simulink library "WECSim_Lib_2019b"  (R2019b)
settings: Solver=ode45  StartTime=0.0  StopTime=10.0  RelTol=1e-3  EnableMultiTasking=on
undefined symbols (not defined in the file or in its folder): body, constraint, mooring, pto, simu, waves, X, Y, Z
libraries: nesl_utility x125, sm_lib x106, $bdroot x16, vrlib x2
(part 9 of 9)

== matlab function WECSim_Lib_2019b/Body Elements/Rigid Body/Hydrodynamic Body/Wave Diffraction and Excitation Force Calculation/Nonlinear FK Force Variant Subsystem/With Nonlinear FroudeKrylov Force/Diffraction and Excitation Forces ==
  data: x input; elv input; center input; f output; tnorm input; area input; rho input; g input; cg input; AH input; w input; dw input; wDepth input; deepWaterWave input; k input; typeNum input; t input; phaseRand input; wp output; wpMeanFS output
function [f, wp, wpMeanFS]  = nonFKForce(x,elv,center,tnorm,area,rho,g,cg,AH,w,dw,wDepth,deepWaterWave,k,typeNum,t,phaseRand)
% Function to calculate the wave excitation force and moment on a
% triangulated surface. The nonlinear excitation forces are calculated by
% intergrating the pressure over the triangulated surface and subtracting
% the linear excitation force (this is added back in later):
%    F_exc_nonlinear = F_exc_total - F_exc_linear
% NOTE: This function assumes that the STL file is imported with its CG at 0,0,0

% Logic to calculate nonFKForce at reduced sample time
[f, wp, wpMeanFS] = calc_force(x,elv,center,tnorm,area,rho,g,cg,AH,w,dw,wDepth,deepWaterWave,k,typeNum,t,phaseRand);
end

function [f, wp, wpMeanFS]  = calc_force(x,elv,center,tnorm,area,rho,g,cg,AH,w,dw,wDepth,deepWaterWave,k,typeNum,t,phaseRand)
% Function to apply translation and rotation, and calculate forces.

% Compute new tri coords after cog rotation and translation
centerMeanFS = offsetXYZ(center,cg);
avMeanFS     = tnorm .* [area area area];

% Compute new tri coords after cog rotation and translation
center = rotateXYZ(center,[1 0 0],x(4));
center = rotateXYZ(center,[0 1 0],x(5));
center = rotateXYZ(center,[0 0 1],x(6));
center = offsetXYZ(center,x);
center = offsetXYZ(center,cg);
% Compute new normal vectors coords after cog rotation and translation
tnorm = rotateXYZ(tnorm,[1 0 0],x(4));
tnorm = rotateXYZ(tnorm,[0 1 0],x(5));
tnorm = rotateXYZ(tnorm,[0 0 1],x(6));

% Copute area vectors
av = tnorm .* [area area area];

% Calculate the free surface
wpMeanFS=pDis(centerMeanFS,       0,AH,w,dw,wDepth,deepWaterWave,t,k,phaseRand,typeNum,rho,g);
wp      =pDis(center      ,     elv,AH,w,dw,wDepth,deepWaterWave,t,k,phaseRand,typeNum,rho,g);

% Calculate forces
f_linear   =FK(centerMeanFS,       cg,avMeanFS,wpMeanFS);
f_nonLinear=FK(center      ,x(1:3)+cg,av      ,wp      );
f = f_nonLinear-f_linear;
end

function f=pDis(center,elv,AH,w,dw,wDepth,deepWaterWave,t,k,phaseRand,typeNum,rho,g)
% Function to calculate pressure distribution
f = zeros(length(center(:,3)),1);
z=zeros(length(center(:,1)),1);
if typeNum <10
elseif typeNum <20
    f = rho.*g.*AH(1).*cos(k(1).*center(:,1)-w(1)*t);
    if deepWaterWave == 0
        z=(center(:,3)-elv).*wDepth./(wDepth+elv);
        f = f.*(cosh(k(1).*(z+wDepth))./cosh(k(1)*wDepth));
    else
        z=(center(:,3)-elv);
        f = f.*exp(k(1).*z);
    end
elseif typeNum <30
    for i=1:length(AH)
        if deepWaterWave == 0 && wDepth <= 0.5*pi/k(i)
            z=(center(:,3)-elv).*wDepth./(wDepth+elv);
            f_tmp = rho.*g.*sqrt(AH(i)*dw(i)).*cos(k(i).*center(:,1)-w(i)*t-phaseRand(i));
            f = f + f_tmp.*(cosh(k(i).*(z+wDepth))./cosh(k(i).*wDepth));
        else
            z=(center(:,3)-elv);
            f_tmp = rho.*g.*sqrt(AH(i)*dw(i)).*cos(k(i).*center(:,1)-w(i)*t-phaseRand(i));
            f = f + f_tmp.*exp(k(i).*z);
        end
    end
end
f(z>0)=0;
end

function f = FK(center,instcg,av,wp)
% Function to calculate the force and moment about the cog due to Froude-Krylov pressure
f = zeros(6,1);

% Calculate the hydrostatic pressure at each triangle center
pressureVect = [wp wp wp].*-av;

% Compute force about cog
f(1:3) = sum(pressureVect);

% Compute moment about cog
tmp1 = ones(length(center(:,1)),1);
tmp2 = tmp1*instcg';
center2cgVec = center-tmp2;

f(4:6)= sum(cross(center2cgVec,pressureVect));
end

== matlab function WECSim_Lib_2019b/Body Elements/Rigid Body/Hydrodynamic Body/Wave Radiation Forces Calculation/SS CI and Constant-Damping-CoeVariant Subsystem/Convolution Integral Calculation/MATLAB Function1 ==
  data: velocity input; F_FM output; IRKB input; CTTime input
function F_FM = ConvolutionIntegral_interp(velocity, IRKB, CTTime)
%#codegen
% Function to calculate convolution integral. velocity is the only dynamic input.
% IRKB, nDOF and CTTime do not change with time.
%
% Dimensions:
% nDOF = the body's number of degrees of freedom = body.dof
% LDOF = radiating dofs from all bodies (6*Nbodies)
% nt = length of CTTime (simu.CITime / simu.dtCTTime)
%
% Paramters:
%     velocity : float [LDOF]
%         The current velocities of all bodies 
%         e.g. 6 for 1 body, 12 for 2 bodies and B2B on
% 
%     IRKB : float [nt nDOF LDOF]
%         The body's interpolated IRF, as calculated in irfInfAddedMassAndDamping
% 
%     CTTime : float [nt]
%         All CI times
%
% Returns:
%     F_FM : float [nDOF,1]

% define persistent variables to track velocity_history over time. Others are
% persistent so that the static values only need be calculated once.
interp_factor = 1;
persistent velocity_history IRKB_interp CTTime_interp;

% If this is the first time step (i.e. velocity_history is empty), 
% define the persistent variables.
if isempty(velocity_history) 
    CTTime_interp  = CTTime(1:interp_factor:end);         % [nt] interpolate CTTime if interpolation timestep ~= 1
    velocity_history = zeros(length(CTTime_interp),length(velocity)); % [nt LDOF]
    irkb_tmp    = IRKB(1:interp_factor:end, :, :);     % [nt nDOF LDOF] interpolate IRKB if interpolation timestep ~= 1
    IRKB_interp = permute(irkb_tmp,[1 3 2]); % permute to [nt LDOF nDOF]
end 

% shift velocity_history to set the first column as the current velocity
velocity_history = circshift(velocity_history, 1, 1); % shift velocity_history by 1 in the time dimension for the new time step
velocity_history(1,:) = velocity(:)';                 % [nt LDOF], fill first row with current velocity

% Multiply velocity_history and IRKB
time_series = bsxfun(@times, IRKB_interp, velocity_history); % [nt LDOF nDOF], multiply velocity_history and K_r for CI integral

% sum the effects of all radiating dofs (LDOF) for each time and motion dof (nDOF)
tmp_s = squeeze(sum(time_series,2)); % [nt nDOF]
F_FM = squeeze(trapz(CTTime_interp,tmp_s,1)); % integrate to get the wave radiation force, [nDOF, 1]

end

== matlab function WECSim_Lib_2019b/Body Elements/Rigid Body/Hydrodynamic Body/nonLinYaw force transforms/nonLinYaw force transforms ==
  data: yawNonLin input; F_Excitation output; dispGlobal input; F_RadiationDampingLocal input; F_AddedMassLocal input; F_ExcitationLocal input; F_RadiationDamping output; F_RestoringLocal input; F_AddedMass output; F_Restoring output
function [F_Excitation, F_RadiationDamping, F_AddedMass, F_Restoring] = fYawTransforms(yawNonLin, dispGlobal, F_RadiationDampingLocal, F_AddedMassLocal, F_ExcitationLocal, F_RestoringLocal)
if yawNonLin ==1
    % transform force vectors from local frame to global frame
    rotMatYaw = [cos(dispGlobal(6)), -sin(dispGlobal(6)), 0;
                 sin(dispGlobal(6)),  cos(dispGlobal(6)), 0;
                                  0,                   0, 1];

    F_RadiationDamping = [rotMatYaw*F_RadiationDampingLocal(1:3); rotMatYaw*F_RadiationDampingLocal(4:6)];
    F_AddedMass = [rotMatYaw*F_AddedMassLocal(1:3); rotMatYaw*F_AddedMassLocal(4:6)];
    F_Excitation = [rotMatYaw*F_ExcitationLocal(1:3); rotMatYaw*F_ExcitationLocal(4:6)];
    F_Restoring = [rotMatYaw*F_RestoringLocal(1:3); rotMatYaw*F_RestoringLocal(4:6)];
else
    F_RadiationDamping = F_RadiationDampingLocal;
    F_AddedMass = F_AddedMassLocal;
    F_Excitation = F_ExcitationLocal;
    F_Restoring = F_RestoringLocal;
end
end

== matlab function WECSim_Lib_2019b/Body Elements/Rigid Body/Hydrodynamic Body/Wave Diffraction and Excitation Force Calculation/Linear Wave Excitation Force Variant Subsystem/Regular Wave NonLinear Yaw/MATLAB Function1 ==
  data: A input; w input; dofGRD input; dirGRD input; fEHRE input; fEHIM input; Fext output; fEHMD input; time input; WaveDir input; Disp input; intThresh input; prevYaw input; relYawLast output; prevCoeffMD input; prevCoeffRE input; prevCoeffIM input; coeffsLastMD output; coeffsLastRE output; coeffsLastIM output
function [Fext,relYawLast,coeffsLastMD,coeffsLastRE,coeffsLastIM] = fcn(A,w,dofGRD,dirGRD,fEHRE,fEHIM, fEHMD,time,WaveDir,Disp, intThresh, prevYaw, prevCoeffMD, prevCoeffRE, prevCoeffIM)
%#codegen
% Fext is the excitation force output, relYawLast is the angle of relative
% yaw at which that last interpolation was performed. If the current
% relative yaw angle - last interpolated > threshold, the interpolation is
% performed again. To interpolate every time step, let threshold=0. 

%initialize outputs
Fext = zeros(1,6);
relYawLast=0;
coeffsLastMD=zeros(length(w),6); % should be (1,6) for regular waves
coeffsLastRE=zeros(length(w),6);
coeffsLastIM=zeros(length(w),6);

for ii=1:length(WaveDir) % should be length=1 for regular waves
    relYaw=WaveDir(ii)-(Disp(6).*180/pi); % relative yaw angle, convert to deg
   
     % compare relYaw to available WaveDir data
        if relYaw>max(dirGRD(1,:)) % handle interpolation out of BEM range by wrapping other bound
            [~,idx]=min(dirGRD,[],2); % 
            dirGRD(:,idx)=dirGRD(:,idx)+360;
            [dirGRD,I]=sort(dirGRD,2); % grid must be in ascending order
            
        elseif relYaw<min(dirGRD(1,:))
            [~,idx]=max(dirGRD,[],2); % 
            dirGRD(:,idx)=dirGRD(:,idx)-360;
            [dirGRD,I]=sort(dirGRD,2); % grid must be in ascending order
        else
            I=1:length(dirGRD(1,:));
        end
        
    if abs(relYaw-prevYaw)>intThresh && min(abs(relYaw-dirGRD(1,:)))>intThresh% interpolate for nonlinear yaw 
       
        % performs 1D interpolation in wave direction
        fExtMDint=interpn(dofGRD,dirGRD,fEHMD(:,I(1,:)),dofGRD,relYaw*ones(size(dirGRD)));
        fExtREint=interpn(dofGRD,dirGRD,fEHRE(:,I(1,:)),dofGRD,relYaw*ones(size(dirGRD)));
        fExtIMint=interpn(dofGRD,dirGRD,fEHIM(:,I(1,:)),dofGRD,relYaw*ones(size(dirGRD)));
        
        fExtMDint=fExtMDint(:,1).';
        fExtREint=fExtREint(:,1).';
        fExtIMint=fExtIMint(:,1).';
                
        relYawLast=relYaw;
        coeffsLastMD=fExtMDint;
        coeffsLastRE=fExtREint;
        coeffsLastIM=fExtIMint;
  
   elseif min(abs(relYaw-dirGRD(1,:)))>intThresh % significant yaw is present, but close to previous value
        fExtMDint=prevCoeffMD;
        fExtREint=prevCoeffRE;
        fExtIMint=prevCoeffIM;
        
        relYawLast=prevYaw;
        coeffsLastMD=prevCoeffMD;
        coeffsLastRE=prevCoeffRE;
        coeffsLastIM=prevCoeffIM;
              
    else    % significant yaw may be is present, but nearby BEM calculated data
        [~,idx]=min(abs(relYaw-dirGRD(1,:)));
        fExtMDint=fEHMD(:,I(1,idx)).'; % maintains dimensional consistency
        fExtREint=fEHRE(:,I(1,idx)).';
        fExtIMint=fEHIM(:,I(1,idx)).';
     
        relYawLast=dirGRD(1,idx); % indices of dirGRD have already been resorted
        coeffsLastMD=fExtMDint;
        coeffsLastRE=fExtREint;
        coeffsLastIM=fExtIMint;
    end

    % regular wave excitation equation (with mean drift)
    Fext = fExtMDint*A^2 + A*fExtREint*cos(w*time)- A*fExtIMint*sin(w*time);
    

end

== matlab function WECSim_Lib_2019b/Body Elements/Rigid Body/Hydrodynamic Body/Kinematic Transforms/No B2B/nonLinYaw Kinematic transforms ==
  data: yawNonLin input; dispLoc output; dispGlobal input; velGlobal input; accGlobal input; velLoc output; accLoc output
function [dispLoc, velLoc, accLoc] = kinYawTransform(yawNonLin, dispGlobal, velGlobal, accGlobal)
if yawNonLin == 1
    % rotate kinematics to 'zero' the yaw displacement (in order to
    % calculate F_RadiationDamping, F_AddedMass and F_Restoring in the
    % local frame).
    rotMatYaw = [cos(dispGlobal(6)), -sin(dispGlobal(6)), 0;
                 sin(dispGlobal(6)),  cos(dispGlobal(6)), 0;
                                  0,                   0, 1];

    rotMatYawTranspose = rotMatYaw.';
    rotMatGlobal = eulXYZ2RotMat(dispGlobal(4), dispGlobal(5), dispGlobal(6));
    rotMatLoc = rotMatYawTranspose*rotMatGlobal;

    [phiLoc, thetaLoc, psiLoc] = rotMatXYZ2Eul(rotMatLoc);
    dispLoc = [rotMatYawTranspose*dispGlobal(1:3); phiLoc; thetaLoc; psiLoc];
    velLoc = [rotMatYawTranspose*velGlobal(1:3); rotMatYawTranspose*velGlobal(4:6)];
    accLoc = [rotMatYawTranspose*accGlobal(1:3); rotMatYawTranspose*accGlobal(4:6)];
else
    dispLoc = dispGlobal;
    velLoc = velGlobal;
    accLoc = accGlobal;
end
end

== matlab function WECSim_Lib_2019b/Body Elements/Flex Body/Wave Diffraction and Excitation Force Calculation/Wave Diffraction and Excitation Force Calculation/Nonlinear FK Force Variant Subsystem/With Nonlinear FroudeKrylov Force/Diffraction and Excitation Forces ==
  data: x input; elv input; center input; f output; tnorm input; area input; rho input; g input; cg input; AH input; w input; dw input; wDepth input; deepWaterWave input; k input; typeNum input; t input; phaseRand input; wp output; wpMeanFS output
function [f, wp, wpMeanFS]  = nonFKForce(x,elv,center,tnorm,area,rho,g,cg,AH,w,dw,wDepth,deepWaterWave,k,typeNum,t,phaseRand)
% Function to calculate the wave excitation force and moment on a
% triangulated surface. The nonlinear excitation forces are calculated by
% intergrating the pressure over the triangulated surface and subtracting
% the linear excitation force (this is added back in later):
%    F_exc_nonlinear = F_exc_total - F_exc_linear
% NOTE: This function assumes that the STL file is imported with its CG at 0,0,0

% Logic to calculate nonFKForce at reduced sample time
[f, wp, wpMeanFS] = calc_force(x,elv,center,tnorm,area,rho,g,cg,AH,w,dw,wDepth,deepWaterWave,k,typeNum,t,phaseRand);
end

function [f, wp, wpMeanFS]  = calc_force(x,elv,center,tnorm,area,rho,g,cg,AH,w,dw,wDepth,deepWaterWave,k,typeNum,t,phaseRand)
% Function to apply translation and rotation, and calculate forces.

% Compute new tri coords after cog rotation and translation
centerMeanFS = offsetXYZ(center,cg);
avMeanFS     = tnorm .* [area area area];

% Compute new tri coords after cog rotation and translation
center = rotateXYZ(center,[1 0 0],x(4));
center = rotateXYZ(center,[0 1 0],x(5));
center = rotateXYZ(center,[0 0 1],x(6));
center = offsetXYZ(center,x);
center = offsetXYZ(center,cg);
% Compute new normal vectors coords after cog rotation and translation
tnorm = rotateXYZ(tnorm,[1 0 0],x(4));
tnorm = rotateXYZ(tnorm,[0 1 0],x(5));
tnorm = rotateXYZ(tnorm,[0 0 1],x(6));

% Copute area vectors
av = tnorm .* [area area area];

% Calculate the free surface
wpMeanFS=pDis(centerMeanFS,       0,AH,w,dw,wDepth,deepWaterWave,t,k,phaseRand,typeNum,rho,g);
wp      =pDis(center      ,     elv,AH,w,dw,wDepth,deepWaterWave,t,k,phaseRand,typeNum,rho,g);

% Calculate forces
f_linear   =FK(centerMeanFS,       cg,avMeanFS,wpMeanFS);
f_nonLinear=FK(center      ,x(1:3)+cg,av      ,wp      );
f = f_nonLinear-f_linear;
end

function f=pDis(center,elv,AH,w,dw,wDepth,deepWaterWave,t,k,phaseRand,typeNum,rho,g)
% Function to calculate pressure distribution
f = zeros(length(center(:,3)),1);
z=zeros(length(center(:,1)),1);
if typeNum <10
elseif typeNum <20
    f = rho.*g.*AH(1).*cos(k(1).*center(:,1)-w(1)*t);
    if deepWaterWave == 0
        z=(center(:,3)-elv).*wDepth./(wDepth+elv);
        f = f.*(cosh(k(1).*(z+wDepth))./cosh(k(1)*wDepth));
    else
        z=(center(:,3)-elv);
        f = f.*exp(k(1).*z);
    end
elseif typeNum <30
    for i=1:length(AH)
        if deepWaterWave == 0 && wDepth <= 0.5*pi/k(i)
            z=(center(:,3)-elv).*wDepth./(wDepth+elv);
            f_tmp = rho.*g.*sqrt(AH(i)*dw(i)).*cos(k(i).*center(:,1)-w(i)*t-phaseRand(i));
            f = f + f_tmp.*(cosh(k(i).*(z+wDepth))./cosh(k(i).*wDepth));
        else
            z=(center(:,3)-elv);
            f_tmp = rho.*g.*sqrt(AH(i)*dw(i)).*cos(k(i).*center(:,1)-w(i)*t-phaseRand(i));
            f = f + f_tmp.*exp(k(i).*z);
        end
    end
end
f(z>0)=0;
end

function f = FK(center,instcg,av,wp)
% Function to calculate the force and moment about the cog due to Froude-Krylov pressure
f = zeros(6,1);

% Calculate the hydrostatic pressure at each triangle center
pressureVect = [wp wp wp].*-av;

% Compute force about cog
f(1:3) = sum(pressureVect);

% Compute moment about cog
tmp1 = ones(length(center(:,1)),1);
tmp2 = tmp1*instcg';
center2cgVec = center-tmp2;

f(4:6)= sum(cross(center2cgVec,pressureVect));
end

== matlab function WECSim_Lib_2019b/Body Elements/Rigid Body/Hydrodynamic Body/Kinematic Transforms/With B2B/MATLAB Function ==
  data: yawNonLin input; dispLoc output; dispGlobal input; velGlobal input; accGlobal input; velLoc output; accLoc output; numBody parameter
function [dispLoc, velLoc, accLoc] = kinYawTransform(yawNonLin, dispGlobal, velGlobal, accGlobal, numBody)

% pre-allocate outputs
    dispLoc=zeros(6,1);
    velLoc=zeros(numBody*6,1);
    accLoc=zeros(numBody*6,1);
    
if yawNonLin == 1
    % rotate kinematics to 'zero' the yaw displacement (in order to
    % calculate F_RadiationDamping, F_AddedMass and F_Restoring in the
    % local frame).
            
    rotMatYaw = [cos(dispGlobal(6)), -sin(dispGlobal(6)), 0;
                 sin(dispGlobal(6)),  cos(dispGlobal(6)), 0;
                                  0,                   0, 1];

    rotMatYawTranspose = rotMatYaw.';
    rotMatGlobal = eulXYZ2RotMat(dispGlobal(4), dispGlobal(5), dispGlobal(6));
    rotMatLoc = rotMatYawTranspose*rotMatGlobal;

    [phiLoc, thetaLoc, psiLoc] = rotMatXYZ2Eul(rotMatLoc);
    dispLoc = [rotMatYawTranspose*dispGlobal(1:3); phiLoc; thetaLoc; psiLoc];
   for k=1:length(velGlobal)/6 % loop through each 6-dof body
        velLoc(6*(k-1)+1:6*(k-1)+6) = [rotMatYawTranspose*velGlobal((6*(k-1)+1):(6*(k-1)+3));...
            rotMatYawTranspose*velGlobal((6*(k-1)+4):(6*(k-1)+6))];
        accLoc(6*(k-1)+1:6*(k-1)+6) = [rotMatYawTranspose*accGlobal((6*(k-1)+1):(6*(k-1)+3));...
            rotMatYawTranspose*accGlobal((6*(k-1)+4):(6*(k-1)+6))];
    end
else
    dispLoc = dispGlobal;
    velLoc = velGlobal;
    accLoc = accGlobal;
end
end

== matlab function WECSim_Lib_2019b/Body Elements/Rigid Body/Hydrodynamic Body/Morison Element and ViscousDampingForceCalculation/Morison Element Variant Subsystem/Morison Element On/Regular Wave Morison Force/MATLAB Function ==
  data: z input; f output; r input; Vel input; Accel input; Disp input; Area input; Cd input; Vol input; Ca input; Time input; rho input; waveDir input; waterDepth input; k input; w input; A input; rampTime input; g input; currentSpeed input; currentDirection input; currentDepth input; currentOption input; simuMorison input
function f = fcn(z,r,Vel,Accel,Disp,Area,Cd,Vol,Ca,Time,rho,waveDir,waterDepth,k,w,A,rampTime,g,currentSpeed,currentDirection,currentDepth,currentOption,simuMorison)
% This function calculates the Morison element force for the regular wave
% case.
[rr,~]=size(r);
FMt = zeros(rr,6);
for ii = 1:rr
    % Calculate Rotation Matrix
    RotMax      = [cos(Disp(5))*cos(Disp(6)) , cos(Disp(4))*sin(Disp(6)) + sin(Disp(4))*sin(Disp(5))*cos(Disp(6)) , sin(Disp(4))*sin(Disp(6)) - cos(Disp(4))*sin(Disp(5))*sin(Disp(6));...
                   -cos(Disp(5))*sin(Disp(6)), cos(Disp(4))*cos(Disp(6)) -  sin(Disp(4))*sin(Disp(5))*sin(Disp(6)), sin(Disp(4))*cos(Disp(6)) + cos(Disp(4))*sin(Disp(5))*sin(Disp(6));...
                   sin(Disp(5))              , -sin(Disp(4))*cos(Disp(5))                                         , cos(Disp(4))*cos(Disp(5))                                        ];
    % Rotate Cartesian
    rRot        = mtimes(RotMax,r(ii,:).')';
    Dispt       = [Disp(1),Disp(2),Disp(3)];
    ShiftCg     = Dispt + rRot;
    zRot        = mtimes(RotMax,z(ii,:)')';
    % Update translational and rotational velocity
    % w refers to \omega = rotational velocity
    Velt        = [Vel(4),Vel(5),Vel(6)];
    wxr         = cross(Velt,r(ii,:));
    %
    switch currentOption
        case 0
            currentSpeedDepth = currentSpeed;
        case 1
            if ShiftCg(3) > -currentDepth
                currentSpeedDepth = currentSpeed*(1 + ShiftCg(3)/currentDepth)^(1/7);
            else
                currentSpeedDepth = 0;
            end
        case 2
            if ShiftCg(3) > -currentDepth
                currentSpeedDepth = currentSpeed*(1 + ShiftCg(3)/currentDepth);
            else
                currentSpeedDepth = 0;
            end
        otherwise
            currentSpeedDepth = 0;
    end
    % Ramp Time
    if Time <= rampTime
        curramp     = currentSpeedDepth*(1 + cos(pi + pi/rampTime*Time))/2;
    else
        curramp     = currentSpeedDepth;
    end
    %Vel should be a column vector
    Vel2            = [Vel(1),Vel(2),Vel(3)] + wxr + [curramp*cosd(currentDirection),curramp*sind(currentDirection),0];
    % Update translational and rotational acceleration
    % dotw refers to \dot{\omega} = rotational acceleration
    Accelt          = [Accel(4),Accel(5),Accel(6)];
    dotwxr          = cross(Accelt,r(ii,:));
    wxwxr           = cross(Velt,wxr);
    Accel2          = [Accel(1),Accel(2),Accel(3)] + dotwxr + wxwxr;
    %% Calculate Orbital Velocity
    waveDirRad      = waveDir*pi/180;
    phaseArg        = w*Time - k*(ShiftCg(1)*cos(waveDirRad) + ShiftCg(2)*sin(waveDirRad));
    % Vertical Variation
    kh              = k*waterDepth;    
    kz              = k*ShiftCg(3);
    if kh > pi  % Deep water wave
        coeffHorz   = exp(kz);
        coeffVert   = coeffHorz;
    else        % Shallow & Intermediate Depth
        coeffHorz   = cosh(kz + kh)/cosh(kh);
        coeffVert   = sinh(kz + kh)/cosh(kh);
    end
    % Ramp Time
    if Time <= rampTime
        ramp        = (A/2)*(1 + cos( pi + pi/rampTime*Time));
    else
        ramp        = A;
    end
    % Orbital Velocity
    uV              =  ramp*coeffHorz*cos(phaseArg)*g*k*(1/w)*cos(waveDirRad);
    vV              =  ramp*coeffHorz*cos(phaseArg)*g*k*(1/w)*sin(waveDirRad);
    wV              = -ramp*coeffVert*sin(phaseArg)*g*k*(1/w);
    fluidV          = [uV, vV, wV];
    % Orbital Acceleration
    uA              = -ramp*coeffHorz*sin(phaseArg)*g*k*cos(waveDirRad);
    vA              = -ramp*coeffHorz*sin(phaseArg)*g*k*sin(waveDirRad);
    wA              = -ramp*coeffVert*cos(phaseArg)*g*k;
    fluidA          = [uA, vA, wA];
    if simuMorison == 2
        %% Decompose Fluid Velocity
        % Tangential Velocity
        vT          = ((dot(zRot,fluidV))/(norm(zRot)^2))*zRot;
        % Normal Velocity
        vN          = fluidV-vT;
        %% Decompose Fluid Acceleration
        AT          = ((dot(zRot,fluidA))/(norm(zRot)^2))*zRot;
        % Normal Acceleration
        AN          = fluidA-AT;
        %% Decompose Body Velocity
        % Tangential Velocity
        Vel2T       = ((dot(zRot,Vel2))/(norm(zRot)^2))*zRot;
        % Normal Velocity
        Vel2N       = Vel2-Vel2T;
        %% Decompose Body Acceleration
        Accel2T     = ((dot(zRot,Accel2))/(norm(zRot))^2)*zRot;
        % Normal Acceleration
        Accel2N     = Accel2-Accel2T;
        %% Morison Equation
        % Forces from velocity drag
        FdN         = (1/2)*rho*Cd(ii,1)*Area(ii,1)*(vN-Vel2N)*norm(vN-Vel2N);    
        FdT         = (1/2)*rho*Cd(ii,2)*Area(ii,2)*(vT-Vel2T)*norm(vT-Vel2T);
        Fd          = FdT + FdN;
        % Forces from body acceleration inertia on the Morison Element
        FiN         = rho*Vol(ii,:)*Ca(ii,1)*(AN - Accel2N);
        FiT         = rho*Vol(ii,:)*Ca(ii,2)*(AT - Accel2T);
        Fbi         = FiN + FiT;
        % Forces from fluid acceleration inertia on the Morison Element
        Ffi         = rho*Vol(ii,:)*(fluidA);
        % Summation of inertial forces on the Morison Element
        Fi          = Ffi + Fbi;
        % Total Force from the Morison Element
        F           = Fi + Fd;
    else
        %% Added inertia and drag forces
        areaRot     = abs(mtimes(Area(ii,:),RotMax));
        CdRot       = mtimes(abs(Cd(ii,:)),RotMax);
        CaRot       = abs(mtimes(Ca(ii,:),RotMax));
        % Forces from velocity drag
        uVdiff      = uV - Vel2(1); FxuV = (1/2)*abs(uVdiff)*uVdiff*rho*CdRot(1)*areaRot(1);
        vVdiff      = vV - Vel2(2); FxvV = (1/2)*abs(vVdiff)*vVdiff*rho*CdRot(2)*areaRot(2);
        wVdiff      = wV - Vel2(3); FxwV = (1/2)*abs(wVdiff)*wVdiff*rho*CdRot(3)*areaRot(3);
        % Forces from body acceleration inertia
        uAdiff      = uA - Accel2(1); FxuA = uAdiff*rho*Vol(ii,:)*CaRot(1);
        vAdiff      = vA - Accel2(2); FxvA = vAdiff*rho*Vol(ii,:)*CaRot(2);
        wAdiff      = wA - Accel2(3); FxwA = wAdiff*rho*Vol(ii,:)*CaRot(3);
        % Forces from fluid acceleration inertia
        FxuAf       = uA*Vol(ii,:)*rho;
        FxvAf       = vA*Vol(ii,:)*rho;
        FxwAf       = wA*Vol(ii,:)*rho;
        % Total Force from the Morison Element
        F           = [FxuV + FxuA + FxuAf,...
                       FxvV + FxvA + FxvAf,...
                       FxwV + FxwA + FxwAf];
    end
    % Determine if the Morison Element point of application goes above the
    % mean water line and does not consider the local surface elevation.
    if ShiftCg(3) > 0
        F           = [0, 0, 0];
        M           = [0, 0, 0];
        FMt(ii,:)   = [F,M];
    else
        % Calculate the moment about the center of gravity for each Morison Element
        M           = cross(rRot,F);
        FMt(ii,:)   = [F,M];
    end
end
f      = 0.*Vel;
f(1:6) = [sum(FMt(:,1));sum(FMt(:,2));sum(FMt(:,3));sum(FMt(:,4));sum(FMt(:,5));sum(FMt(:,6))];
end
